simulink model "MTi680_SerialReadout"  (R2023b)
settings: Solver=FixedStepAuto  StartTime=0.0  StopTime=inf  RelTol=1e-3
libraries: slrealtimeseriallib x3
settings Model: Creator=matlab.cut  LastModifiedBy=matlab.cut
settings SolverCC: ConcurrentTasks=on  PositivePriorityOrder=on
settings OptimizationCC: BlockReduction=off  OptimizeBlockIOStorage=off
settings DebuggingCC: TasksWithSamePriorityMsg=none
settings HardwareCC: ProdBitPerLong=64  ProdLongLongMode=on  ProdHWDeviceType=Intel->x86-64 (Linux 64)
settings RTWCC: Description=Simulink Real-Time  SystemTargetFile=slrealtime.tlc  TemplateMakefile=slrealtime_default_tmf  Toolchain=Simulink Real-Time Toolchain  BuildConfiguration=Faster Runs  CodeExecutionProfiling=on  TargetLang=C++

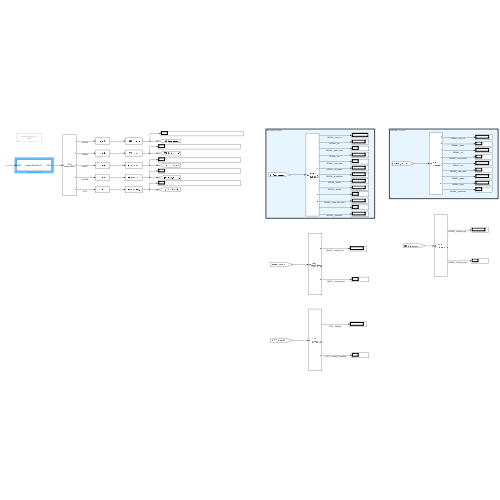
[thumbnail: Simulink's stored preview of the top-level diagram]
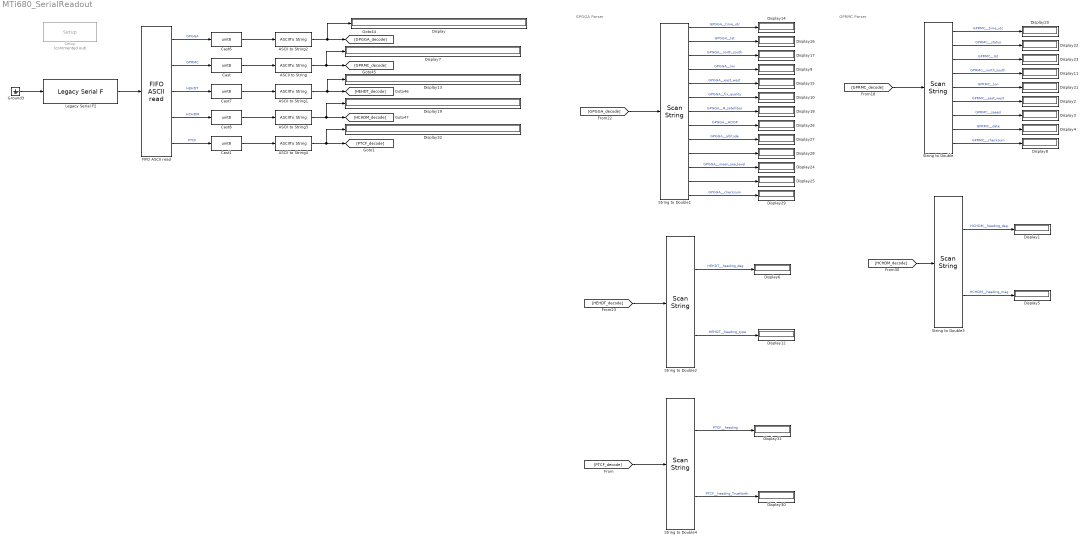
== system MTi680_SerialReadout ==
  note: GPGGA Parser
  note: GPRMC Parser
  ASCII to String{,1..4} (5 alike) : ASCIIToString
  Cast{,1,6..8} (5 alike) : DataTypeConversion  OutDataTypeStr=uint8  SaturateOnIntegerOverflow=off  RndMeth=Floor
  Display{,1..32} (33 alike) : Display
  FIFO ASCII read : slrealtimeseriallib/FIFO ASCII read  header={'$GPGGA', '$GPRMC','$HEHDT','$HCHDM','$PTCF'}  term=[13 10]  hold=Hold last output if no new data  enable=off  maxsize=1024  outputtype=8 bit uint null terminated  sampletime=-1
  Ground3 : Ground
  Legacy Serial F2 : slrealtimeseriallib/Mainboard/Legacy Serial F  port=Legacy Serial Port 1  baud=115200  width=8  nstop=1  parity=None  ctsmode=off  fifosize=1024  idtype=8 bit uint null terminated  sampletime=1e-3
  Setup : slrealtimeseriallib/Mainboard/Setup  Commented=on  port=Legacy Serial Port 1  baud=115200  width=8  nstop=1  parity=None  ctsmode=off
  String to Double : ScanString  Format="\"$GPRMC,%f,%c,%f,%c,%f,%c,%f,,%d,,,%s\""
  String to Double1 : ScanString  Format="\"$GPGGA,%f,%f,%c,%f,%c,%d,%d,%f,%f,%c,%g,%c,,%f\""
  String to Double2 : ScanString  Format="\"$HEHDT,%f,%c\""
  String to Double3 : ScanString  Format="\"$HCHDM,%f,%c\""
  String to Double4 : ScanString  Format="\"$PTCF,%f,%c\""
  wires:
  String to Double3/1 -> Display1/1  "HCHDM__heading_deg"
  String to Double3/2 -> Display5/1  "HCHDM__heading_mag"
  Cast8/1 -> ASCII to String3/1
  ASCII to String1/1 -> Display13/1, [HEHDT_decode]
  String to Double1/1 -> Display14/1  "GPGGA__time_utc"
  String to Double1/8 -> Display26/1  "GPGGA__HDOP"
  String to Double1/2 -> Display16/1  "GPGGA__lat"
  String to Double1/4 -> Display9/1  "GPGGA__lon"
  String to Double1/6 -> Display10/1  "GPGGA__fix_quality"
  String to Double1/13 -> Display29/1  "GPGGA__checksum"
  String to Double1/11 -> Display24/1  "GPGGA__mean_sea_level"
  String to Double1/9 -> Display27/1  "GPGGA__altitude"
  String to Double1/7 -> Display18/1  "GPGGA__#_satellites"
  Ground3/1 -> Legacy Serial F2/1
  [GPRMC_decode] -> String to Double/1
  String to Double2/1 -> Display6/1  "HEHDT__heading_deg"
  Cast7/1 -> ASCII to String1/1
  [HEHDT_decode] -> String to Double2/1
  Legacy Serial F2/1 -> FIFO ASCII read/1
  ASCII to String/1 -> Display7/1, [GPRMC_decode]
  Cast/1 -> ASCII to String/1
  FIFO ASCII read/1 -> Cast6/1  "GPGGA"
  String to Double/8 -> Display4/1  "GPRMC__date"
  String to Double/4 -> Display11/1  "GPRMC__north_south"
  String to Double/3 -> Display23/1  "GPRMC__lat"
  String to Double1/5 -> Display15/1  "GPGGA__east_west"
  String to Double1/12 -> Display25/1
  String to Double/2 -> Display22/1  "GPRMC__status"
  String to Double/5 -> Display21/1  "GPRMC__lon"
  ASCII to String2/1 -> Display/1, [GPGGA_decode]
  String to Double/9 -> Display8/1  "GPRMC__checksum"
  String to Double/6 -> Display2/1  "GPRMC__east_west"
  String to Double1/3 -> Display17/1  "GPGGA__north_south"
  FIFO ASCII read/2 -> Cast/1  "GPRMC"
  ASCII to String3/1 -> Display19/1, [HCHDM_decode]
  String to Double2/2 -> Display12/1  "HEHDT__heading_type"
  FIFO ASCII read/3 -> Cast7/1  "HEHDT"
  String to Double/1 -> Display20/1  "GPRMC__time_utc"
  FIFO ASCII read/4 -> Cast8/1  "HCHDM"
  String to Double/7 -> Display3/1  "GPRMC__speed"
  [GPGGA_decode] -> String to Double1/1
  [HCHDM_decode] -> String to Double3/1
  String to Double1/10 -> Display28/1
  Cast6/1 -> ASCII to String2/1
  String to Double4/1 -> Display31/1  "PTCF__heading"
  String to Double4/2 -> Display30/1  "PTCF__heading_TrueNorth"
  [PTCF_decode] -> String to Double4/1
  ASCII to String4/1 -> Display32/1, [PTCF_decode]
  Cast1/1 -> ASCII to String4/1
  FIFO ASCII read/5 -> Cast1/1  "PTCF"
